simulink model "STV_Scalar_test"  (Simulink 7.3)
settings: Solver=ode45  StartTime=0.0  StopTime=10.0  RelTol=1e-3
settings Model: Creator=MD710  LastModifiedBy=MD710
settings DebuggingCC: SaveWithParameterizedLinksMsg=none  SolverPrmCheckMsg=none  MultiTaskDSMMsg=warning  MultiTaskCondExecSysMsg=none  FcnCallInpInsideContextMsg=Enable All  StrictBusMsg=None
settings HardwareCC: TargetHWDeviceType=32-bit Generic
settings RTWCC: IncludeERTFirstTime=on
settings GRTTargetCC: TargetFcnLib=ansi_tfl_tmw.mat

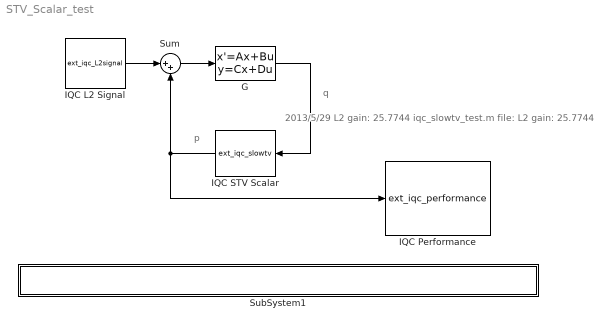
== system STV_Scalar_test ==
  note: q
  note: p
  note: 2013/5/29 L2 gain: 25.7744
      | iqc_slowtv_test.m file:
      | L2 gain: 25.7744
  G : StateSpace  A=[-0.21 -1; 1 0]  B=[0.8;0]  C=[0 1]  D=0
  IQC L2 Signal : M-S-Function  FunctionName=ext_iqc_L2signal  Parameters=sig_size,sam_time,sig_type,tru_time,sig_amp,sig_fre,user_cus  mask(IQC L2 signal(ver:0.1)){sig_size=1, sam_time=0, sig_type=Step, tru_time=10, sig_amp=1, sig_fre=1, user_cus='2*exp(3*t)'}
      mask prompts: sig_size "Signal Dimension:(Default: 1)"; sam_time "Sample Time:(Default: 0)"; sig_type "Signal Type:"; tru_time "Truncation Time:"; sig_amp "Maximum Amplitude:"; sig_fre "Frequency:"; user_cus "Custom:"
      mask help:
      | Important:
      | In IQC procedure step (as commond iqc_gain_tbx, the task is get
      | L2 gain value), regardless of the user to choose which option (ex sine...),
      | here regarded as generalized L2 signal.
      mask StyleString: edit,edit,popup(Step|Square wave|Sine wave|Custom|Random|External),edit,edit,edit,edit
      mask CallbackString: ||iqc_block_cho(gcb,'L2signal_type')||||
      mask TabNameString: Generalized Parameters,Generalized Parameters,Simulink Parameters,Simulink Parameters,Simulink Parameters,Simulink Parameters,Simulink Parameters
      mask Display: plot(0:0.1:10,[sin(0:0.1:6.2) zeros(1,38)])
  IQC Performance : M-S-Function  FunctionName=ext_iqc_performance  Parameters=imp_met,save_lin_com,isiqcbode,fre_ran,uselmitool,lmi_par  mask(IQC Performance(ver:0.1)){imp_met=Only Calculation, save_lin_com=off, isiqcbode=off, fre_ran='', uselmitool=lmilab, lmi_par=''}
      mask prompts: imp_met "Implementation Methods"; save_lin_com "Save the Linear File and Command File"; isiqcbode "Display IQC Bode Figure"; fre_ran "Frequency Range:(Default: empty)"; uselmitool "LMI Tool:"; lmi_par "Parameter:(if empty use define)"
      mask help:
      | Important:
      | In IQC toolbox calculate step (as commond iqc_gain_tbx, the task is get
      | L2 gain value), regardless of the user to connect any signal input(Even if
      | not a signal), here regarded as generalized L2 signal.
      |
      | Example 1: setlmioptions('',[0 200 0 0 777])
      | the block parameter is
      | LMI Tool: lmilab
      | Parameter:
      |        [0 200 0 0 777]
      |
      | Example 2: setlmioptions('yalmip','solver','sdpt3','verbose',1)
      | the block parameter is
      | LMI Tool: yalmip
      | Parameter:
      |        {'solver',sdpt3','verbose',1}
      mask Help:
      | <a href="matlab:doc abst_init_iqc;">abst_init_iqc</a>
      | <a href="matlab:doc setlmioptions;">setlmioptions</a>
      | <a href="matlab:doc iqc_gain_tbx;">iqc_gain_tbx</a>
      mask StyleString: popup(Calculation and Simulation|Only Calculation|Only Simulation),checkbox,checkbox,edit,popup(lmilab|yalmip),edit
      mask CallbackString: iqc_block_cho(gcb,'performance_imp')||iqc_block_cho(gcb,'performance_bodefre')|||
      mask TabNameString: Parameter,Parameter,Parameter,Parameter,LMI Parameter,LMI Parameter
      mask Display: fprintf('In -> Out \n performance \n L2 gain:\n%4.4f',25.7744);
  IQC STV Scalar : M-S-Function  FunctionName=ext_iqc_slowtv  Parameters=upp_bou_dd,pole,upp_bou_d,out_var  mask(IQC STV Scalar(ver:0.1)){upp_bou_dd=0.1, pole=[1 3 5], upp_bou_d=1, out_var=''}
      mask prompts: upp_bou_dd "Upper Bound of The L-inf norm of d(delta)/dt:(Default: 1)"; pole "Pole:(Default [1])"; upp_bou_d "Upper Bound of The L-inf norm of delta:(Default: 1)"; out_var "Output Variable:(Default: empty)"
      mask help:
      | Example: [w,K1,M1,K2,M2]=iqc_slowtv(v,d,a,D)
      | Upper Bound of The L-inf norm of d(delta)/dt:
      |                   d
      | Pole:
      |                  [a]
      | Upper Bound of The L-inf norm of (delta):
      |                   D
      | Output Variable:
      |                  {'K1','M1','K2','M2'}
      mask Help: eval('doc iqc_slowtv')
      mask Display: disp('\fontsize{16}|D^\prime| < k', 'texmode','on')
  SubSystem1 : Subsystem  mask{filename=iqc_slowtv_test.m}
      mask init:
      | x_dir=which(filename);
      | x=x_dir;
      settings: OpenFcn=|
      | x_dir=which('iqc_slowtv_test.m');
      | x=x_dir;
      | edit(x);
      mask Display: disp(['MATLAB file: ' x]);
  Sum : Sum  Inputs=|++
  wires:
  Sum/1 -> G/1
  IQC L2 Signal/1 -> Sum/1
  G/1 -> IQC STV Scalar/1
  IQC STV Scalar/1 -> IQC Performance/1, Sum/2

== system STV_Scalar_test/SubSystem1 ==
